simulink model "BIMUOk"  (R2024b)
settings: Solver=FixedStepAuto  StartTime=0.0  StopTime=10.0  RelTol=1e-3  EnableMultiTasking=on
undefined symbols (not defined in the file): tSystemsTask
libraries: simulink x9
settings Model: DataDictionary=Master_Dictionary.sldd  EnableAccessToBaseWorkspace=off  Creator=thoma  LastModifiedBy=Will
settings OptimizationCC: DefaultParameterBehavior=Inlined  EnhancedBackFolding=on  PassReuseOutputArgsAs=Individual arguments  ZeroExternalMemoryAtStartup=off  ZeroInternalMemoryAtStartup=off  MaxStackSize=8192  OptimizeBlockOrder=speed  DifferentSizesBufferReuse=on  OptimizationCustomize=off  EfficientTunableParamExpr=on
settings DebuggingCC: ParameterTunabilityLossMsg=error
settings HardwareCC: ProdBitPerPointer=32  ProdBitPerSizeT=32  ProdBitPerPtrDiffT=32  ProdLargestAtomicInteger=Long  ProdLargestAtomicFloat=Double  ProdWordSize=32  ProdLongLongMode=on  ProdHWDeviceType=ARM Compatible->ARM Cortex-M
settings SFSimCC: MATLABDynamicMemAlloc=off
settings RTWCC: Description=Embedded Coder  SystemTargetFile=ert.tlc  HardwareBoard=STM32H7xx Based (Single-core)  TemplateMakefile=ert_default_tmf  Toolchain=GNU Tools for ARM Embedded Processors
settings CodeAppCC: ForceParamTrailComments=on  IgnoreCustomStorageClasses=off  OperatorAnnotations=on  SimulinkDataObjDesc=on  SFDataObjDesc=on  InsertBlockDesc=on
settings ERTTargetCC: TargetLangStandard=C99 (ISO)  CodeReplacementLibrary=ARM Cortex-M  ExtModeTransport=3  ExtModeStaticAlloc=on  ExtModeStaticAllocSize=2048  ExtModeMexFile=ext_xcp  ExtModeIntrfLevel=Level2 - Open

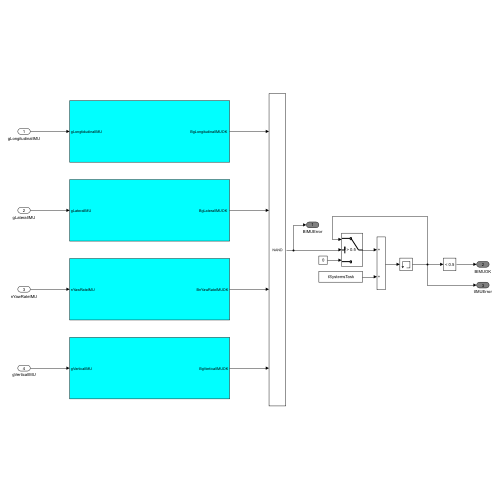
[thumbnail: Simulink's stored preview of the top-level diagram]
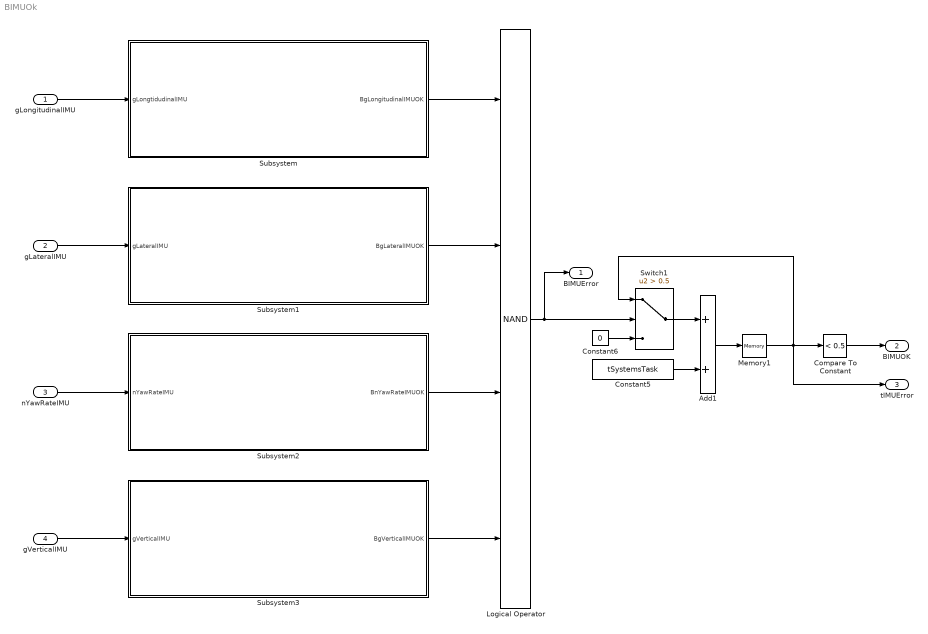
== system BIMUOk ==
  gLongitudinalIMU : Inport  OutDataTypeStr=double
  gLateralIMU : Inport  Port=2  OutDataTypeStr=double
  nYawRateIMU : Inport  Port=3  OutDataTypeStr=double
  gVerticalIMU : Inport  Port=4  OutDataTypeStr=double
  Add1 : Sum
  Compare To Constant : simulink/Logic and Bit Operations/Compare To Constant  relop=<  const=0.5  OutDataTypeStr=boolean
  Constant5 : Constant  Value=tSystemsTask
  Constant6 : Constant  Value=0
  Logical Operator : Logic  Operator=NAND  Inputs=4  AllPortsSameDT=off  OutDataTypeStr=boolean
  Memory1 : Memory  InheritSampleTime=on
  Subsystem : Subsystem
  Subsystem1 : Subsystem
  Subsystem2 : Subsystem
  Subsystem3 : Subsystem
  Switch1 : Switch  Criteria=u2 > Threshold  Threshold=0.5  SaturateOnIntegerOverflow=off  InputSameDT=off
  BIMUError : Outport  OutDataTypeStr=boolean  VectorParamsAs1DForOutWhenUnconnected=off
  BIMUOK : Outport  Port=2  OutDataTypeStr=boolean  VectorParamsAs1DForOutWhenUnconnected=off
  tIMUError : Outport  Port=3  OutDataTypeStr=double  VectorParamsAs1DForOutWhenUnconnected=off
  wires:
  Subsystem1/1("BgLateralIMUOK ") -> Logical Operator/2
  nYawRateIMU/1 -> Subsystem2/1(nYawRateIMU)
  gLateralIMU/1 -> Subsystem1/1(gLateralIMU)
  gVerticalIMU/1 -> Subsystem3/1(gVerticalIMU)
  Subsystem2/1(BnYawRateIMUOK) -> Logical Operator/3
  Subsystem3/1(BgVerticalIMUOK) -> Logical Operator/4
  Subsystem/1("BgLongitudinalIMUOK ") -> Logical Operator/1
  gLongitudinalIMU/1 -> Subsystem/1(gLongtidudinalIMU)
  Logical Operator/1 -> BIMUError/1, Switch1/2
  Add1/1 -> Memory1/1
  Constant6/1 -> Switch1/3
  Constant5/1 -> Add1/2
  Memory1/1 -> tIMUError/1, Compare To Constant/1, Switch1/1
  Switch1/1 -> Add1/1
  Compare To Constant/1 -> BIMUOK/1

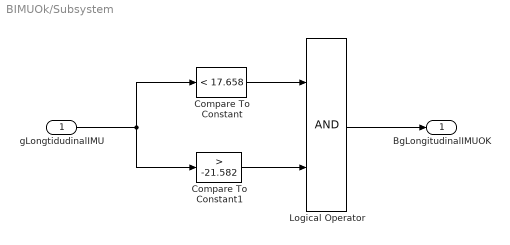
== system BIMUOk/Subsystem ==
  gLongtidudinalIMU : Inport  OutDataTypeStr=double
  Compare To Constant : simulink/Logic and Bit Operations/Compare To Constant  relop=<  const=17.658  OutDataTypeStr=boolean
  Compare To Constant1 : simulink/Logic and Bit Operations/Compare To Constant  relop=>  const=-21.582  OutDataTypeStr=boolean
  Logical Operator : Logic  AllPortsSameDT=off  OutDataTypeStr=boolean
  "BgLongitudinalIMUOK " : Outport  OutDataTypeStr=boolean  VectorParamsAs1DForOutWhenUnconnected=off
  wires:
  Logical Operator/1 -> "BgLongitudinalIMUOK "/1
  Compare To Constant/1 -> Logical Operator/1
  Compare To Constant1/1 -> Logical Operator/2
  gLongtidudinalIMU/1 -> Compare To Constant1/1, Compare To Constant/1

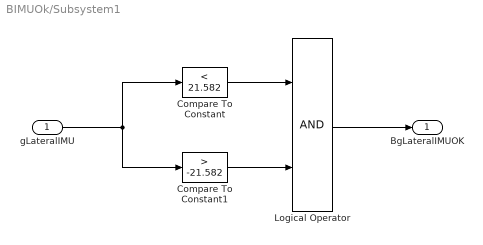
== system BIMUOk/Subsystem1 ==
  gLateralIMU : Inport  OutDataTypeStr=double
  Compare To Constant : simulink/Logic and Bit Operations/Compare To Constant  relop=<  const=21.582  OutDataTypeStr=boolean
  Compare To Constant1 : simulink/Logic and Bit Operations/Compare To Constant  relop=>  const=-21.582  OutDataTypeStr=boolean
  Logical Operator : Logic  AllPortsSameDT=off  OutDataTypeStr=boolean
  "BgLateralIMUOK " : Outport  OutDataTypeStr=boolean  VectorParamsAs1DForOutWhenUnconnected=off
  wires:
  gLateralIMU/1 -> Compare To Constant/1, Compare To Constant1/1
  Compare To Constant1/1 -> Logical Operator/2
  Compare To Constant/1 -> Logical Operator/1
  Logical Operator/1 -> "BgLateralIMUOK "/1

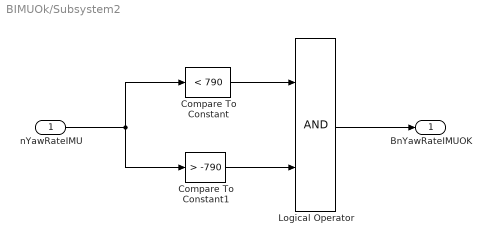
== system BIMUOk/Subsystem2 ==
  nYawRateIMU : Inport  OutDataTypeStr=double
  Compare To Constant : simulink/Logic and Bit Operations/Compare To Constant  relop=<  const=790  OutDataTypeStr=boolean
  Compare To Constant1 : simulink/Logic and Bit Operations/Compare To Constant  relop=>  const=-790  OutDataTypeStr=boolean
  Logical Operator : Logic  AllPortsSameDT=off  OutDataTypeStr=boolean
  BnYawRateIMUOK : Outport  OutDataTypeStr=boolean  VectorParamsAs1DForOutWhenUnconnected=off
  wires:
  Logical Operator/1 -> BnYawRateIMUOK/1
  Compare To Constant/1 -> Logical Operator/1
  Compare To Constant1/1 -> Logical Operator/2
  nYawRateIMU/1 -> Compare To Constant1/1, Compare To Constant/1

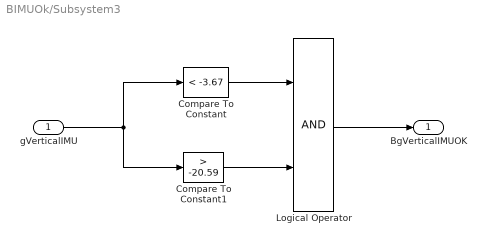
== system BIMUOk/Subsystem3 ==
  gVerticalIMU : Inport  OutDataTypeStr=double
  Compare To Constant : simulink/Logic and Bit Operations/Compare To Constant  relop=<  const=-3.67  OutDataTypeStr=boolean
  Compare To Constant1 : simulink/Logic and Bit Operations/Compare To Constant  relop=>  const=-20.59  OutDataTypeStr=boolean
  Logical Operator : Logic  AllPortsSameDT=off  OutDataTypeStr=boolean
  BgVerticalIMUOK : Outport  OutDataTypeStr=boolean  VectorParamsAs1DForOutWhenUnconnected=off
  wires:
  Logical Operator/1 -> BgVerticalIMUOK/1
  Compare To Constant/1 -> Logical Operator/1
  Compare To Constant1/1 -> Logical Operator/2
  gVerticalIMU/1 -> Compare To Constant1/1, Compare To Constant/1
